simulink model "switchTry"  (Simulink 7.9)
settings: Solver=ode45  StartTime=0.0  StopTime=10.0  RelTol=1e-3
settings Model: Creator=root  LastModifiedBy=root

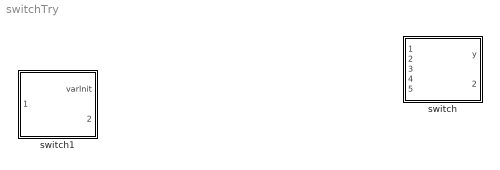
== system switchTry ==
  switch : MATLAB Function  TreatAsAtomicUnit=on
  switch1 : MATLAB Function  TreatAsAtomicUnit=on

== matlab function switch ==
  data: y output double; globalStateOut output double; ActualAngle input double; criticalAngle input double; swingUp input double; LQRcontroller input double; globalState input double
function [y, globalStateOut] = fcn(ActualAngle, criticalAngle, swingUp, LQRcontroller, globalState)
%function y = fcn(swingUp, LQRcontroller, globalState)
%
if (ActualAngle < criticalAngle && globalState == 0)
    y = swingUp;
    %swingOff = 0;
    globalStateOut = 0;
else if (ActualAngle >= criticalAngle || globalState == 1)
    y = LQRcontroller;
    globalStateOut = 1;
    %swingOff = 1;
end
end

== matlab function switch1 ==
  data: varInit output double; varUpdate input double; varUpdated output double
function [varInit, varUpdated] = globalHandler(varUpdate)
%
    if(varUpdate ~= varInit)
        var =  1;
    else
        var = 0;
    end
    if (varUpdate==1)
        varUpdated = 1;
    else
        varUpdated = 0;
    end
end
